simulink model "TrackerMultipleObjects"  (Simulink 8.4)
settings: Solver=FixedStepDiscrete  StartTime=0.0  StopTime=inf  RelTol=1e-3
libraries: instrumentlib x2
settings Model: Creator=Ssubrama  LastModifiedBy=kpetersen
settings OptimizationCC: InitFltsAndDblsToZero=on
settings GRTTargetCC: TargetFcnLib=ansi_tfl_tmw_new.mat

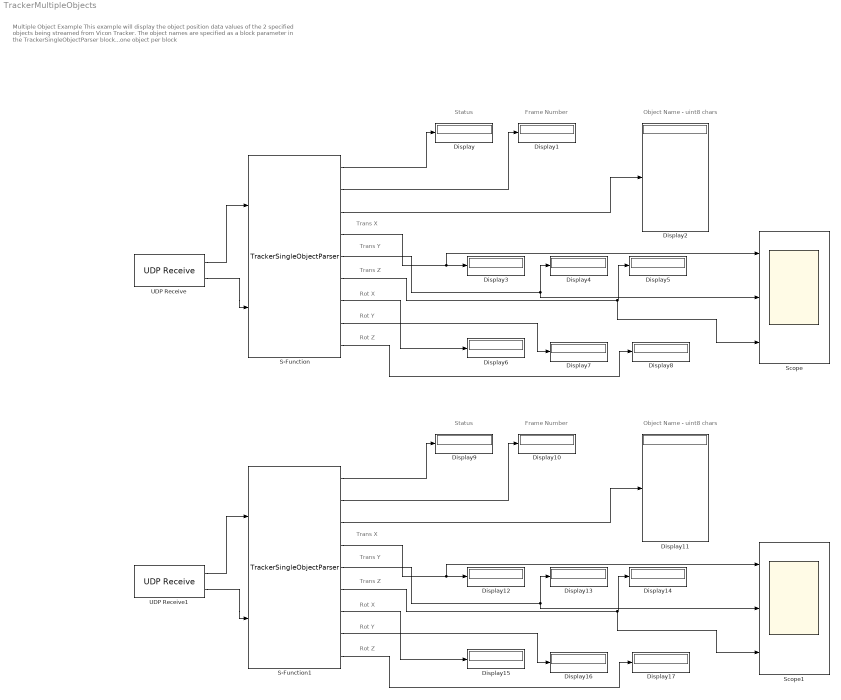
== system TrackerMultipleObjects ==
  note: Rot Z
  note: Rot Y
  note: Rot X
  note: Trans Z
  note: Trans Y
  note: Trans X
  note: Multiple Object Example
      |
      | This example will display the object position data
      | values of the 2 specified objects being streamed from
      | Vicon Tracker.
      |
      | The object names are specified as a block parameter
      | in the TrackerSingleObjectParser block...one object per block
  note: Object Name - uint8 chars
  note: Frame Number
  note: Status
  note: Rot Z
  note: Rot Y
  note: Rot X
  note: Trans Z
  note: Trans Y
  note: Trans X
  note: Object Name - uint8 chars
  note: Frame Number
  note: Status
  Display{,1..17} (18 alike) : Display
  S-Function : S-Function  FunctionName=TrackerSingleObjectParser  Parameters='Object1'  SFunctionModules=TrackerSingleObjectParser  EnableBusSupport=off
      settings: AttributesFormatString=Data Parser
  S-Function1 : S-Function  FunctionName=TrackerSingleObjectParser  Parameters='Object2'  SFunctionModules=TrackerSingleObjectParser  EnableBusSupport=off
      settings: AttributesFormatString=Data Parser
  Scope : Scope  NumInputPorts=3
      settings: YMin=0.4~-4~0.8  YMax=0.8~4~1  MaxDataPoints=200  SampleInput=on  ScrollMode=on
  Scope1 : Scope  NumInputPorts=3
      settings: YMin=0.4~-4~0.8  YMax=0.8~4~1  MaxDataPoints=200  SampleInput=on  ScrollMode=on
  UDP Receive : instrumentlib/UDP Receive  Priority=3  Host=localhost  Port=51001  LocalPort=51001  DataSize=256  EnableBlockingMode=off  Timeout=inf  SampleTime=0.01  DataType=uint8  ByteOrder=BigEndian
  UDP Receive1 : instrumentlib/UDP Receive  Priority=3  Host=localhost  Port=51002  LocalPort=51002  DataSize=256  EnableBlockingMode=off  Timeout=inf  SampleTime=0.01  DataType=uint8  ByteOrder=BigEndian
  wires:
  UDP Receive/1 -> S-Function/1
  S-Function/1 -> Display/1
  UDP Receive/2 -> S-Function/2
  S-Function/2 -> Display1/1
  S-Function/3 -> Display2/1
  S-Function/5 -> Display4/1, Scope/2
  S-Function/6 -> Scope/3, Display5/1
  S-Function/7 -> Display6/1
  S-Function/8 -> Display7/1
  S-Function/9 -> Display8/1
  S-Function/4 -> Scope/1, Display3/1
  UDP Receive1/1 -> S-Function1/1
  S-Function1/1 -> Display9/1
  UDP Receive1/2 -> S-Function1/2
  S-Function1/2 -> Display10/1
  S-Function1/3 -> Display11/1
  S-Function1/5 -> Display13/1, Scope1/2
  S-Function1/6 -> Scope1/3, Display14/1
  S-Function1/7 -> Display15/1
  S-Function1/8 -> Display16/1
  S-Function1/9 -> Display17/1
  S-Function1/4 -> Scope1/1, Display12/1
